simulink model "rawread_slx"  (R2023b)
settings: Solver=FixedStepAuto  StartTime=0.0  StopTime=0  RelTol=1e-3
values from neighbouring files (symbols this model uses):
  m = zeros(size(cfa, 1), 1)    [do.m]
  n = zeros(size(cfa, 2), 1)    [do.m]
  wb = rawInfo.ColorInfo.CameraAsTakenWhiteBalance    [do.m]
  wbcam = rawInfo.ColorInfo.D65WhiteBalance    [do.m]
  xyz = rawInfo.ColorInfo.CameraToXYZ    [do.m]
undefined symbols (not defined in the file or in its folder): gray
settings Model: ParamWorkspaceSource=ReferencedWorkspace  Creator=49176  LastModifiedBy=vithani
settings SolverCC: AllowMultiTaskInputOutput=on  ConcurrentTasks=on  AutoInsertRateTranBlk=on
settings SFSimCC: SimTargetLang=C++

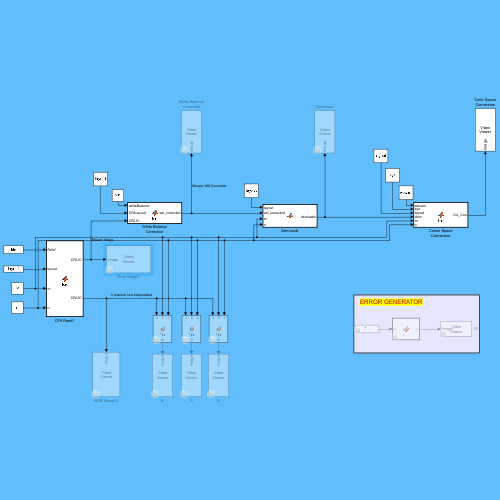
[thumbnail: Simulink's stored preview of the top-level diagram]
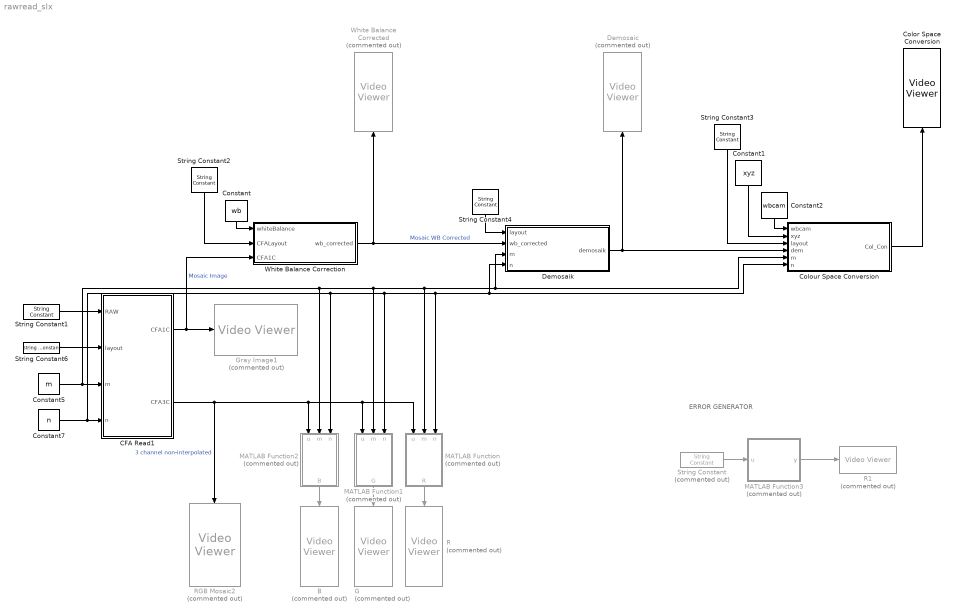
== system rawread_slx ==
  note: ERROR GENERATOR
  B : VideoViewer  Commented=on  colormapValue=gray(256)  FigPos=[1003 1173.33333333333 826.666666666667 737.333333333333]
  CFA Read1 : MATLAB Function  TreatAsAtomicUnit=on
  Color Space Conversion : VideoViewer  colormapValue=gray(256)  FigPos=[771.666666666667 1071.33333333333 884 518]
  Colour Space Conversion : MATLAB Function  TreatAsAtomicUnit=on
  Constant : Constant  Value=wb
  Constant1 : Constant  Value=xyz
  Constant2 : Constant  Value=wbcam
  Constant5 : Constant  Value=m  VectorParams1D=off
  Constant7 : Constant  Value=n  VectorParams1D=off
  Demosaic : VideoViewer  Commented=on  colormapValue=gray(256)  FigPos=[715.666666666667 964 852 619.333333333333]
  Demosaik : MATLAB Function  TreatAsAtomicUnit=on
  G : VideoViewer  Commented=on  colormapValue=gray(256)  FigPos=[819.666666666667 1044.66666666667 714 319.333333333333]
  Gray Image1 : VideoViewer  Commented=on  colormapValue=gray(256)  FigPos=[423 1558.66666666667 1238.66666666667 816.666666666667]
  MATLAB Function : MATLAB Function  Commented=on  TreatAsAtomicUnit=on
  MATLAB Function1 : MATLAB Function  Commented=on  TreatAsAtomicUnit=on
  MATLAB Function2 : MATLAB Function  Commented=on  TreatAsAtomicUnit=on
  MATLAB Function3 : MATLAB Function  Commented=on  TreatAsAtomicUnit=on
  R : VideoViewer  Commented=on  colormapValue=gray(256)  FigPos=[881 962 798.666666666667 486]
  R1 : VideoViewer  Commented=on  colormapValue=gray(256)  FigPos=[881 962 798.666666666667 486]
  RGB Mosaic2 : VideoViewer  Commented=on  colormapValue=gray(256)  FigPos=[924.333333333333 1074.66666666667 930 472]
  String Constant : StringConstant  Commented=on  String=file
  String Constant1 : StringConstant  String=file
  String Constant{2..4,6} (4 alike) : StringConstant  String=layout
  White Balance Corrected : VideoViewer  Commented=on  colormapValue=gray(256)  FigPos=[1323.66666666667 1579.33333333333 958.666666666667 1055.33333333333]
  White Balance Correction : MATLAB Function  TreatAsAtomicUnit=on
  wires:
  CFA Read1/1(CFA1C) -> White Balance Correction/3(CFA1C), Gray Image1/1  "Mosaic Image"
  String Constant1/1 -> CFA Read1/1(RAW)
  CFA Read1/2(CFA3C) -> MATLAB Function/1(u), MATLAB Function1/1(u), MATLAB Function2/1(u), RGB Mosaic2/1  "3 channel non-interpolated"
  MATLAB Function/1(R) -> R/1
  MATLAB Function1/1(G) -> G/1
  MATLAB Function2/1(B) -> B/1
  White Balance Correction/1(wb_corrected) -> White Balance Corrected/1, Demosaik/2(wb_corrected)  "Mosaic WB Corrected"
  Colour Space Conversion/1(Col_Con) -> Color Space Conversion/1
  Constant/1 -> White Balance Correction/1(whiteBalance)
  String Constant2/1 -> White Balance Correction/2(CFALayout)
  Demosaik/1(demosaik) -> Demosaic/1, Colour Space Conversion/4(dem)
  Constant2/1 -> Colour Space Conversion/1(wbcam)
  Constant1/1 -> Colour Space Conversion/2(xyz)
  String Constant3/1 -> Colour Space Conversion/3(layout)
  String Constant4/1 -> Demosaik/1(layout)
  String Constant6/1 -> CFA Read1/2(layout)
  Constant5/1 -> CFA Read1/3(m), MATLAB Function1/2(m), Colour Space Conversion/5(m), Demosaik/3(m), MATLAB Function/2(m), MATLAB Function2/2(m)
  Constant7/1 -> MATLAB Function/3(n), Colour Space Conversion/6(n), Demosaik/4(n), MATLAB Function1/3(n), MATLAB Function2/3(n), CFA Read1/4(n)
  MATLAB Function3/1(y) -> R1/1
  String Constant/1 -> MATLAB Function3/1(u)

== matlab function rawread_slx/CFA Read1 ==
  data: RAW input; CFA1C output; CFA3C output; layout input; m input; n input
function [CFA1C, CFA3C] = fcn(RAW, layout, m, n)

% to mitigate code generation error as limitaion with simulink fcn block
coder.extrinsic("rawread", "rawinfo", "imfinfo","im2uint16");

% global var
a = size(m, 1) ; b = size(n, 1);

% pre-initialising
cfa     = zeros(a, b, "double");
red     = zeros(a, b, "uint16");
blue    = zeros(a, b, "uint16");
green   = zeros(a, b, "uint16");
R       = zeros(a, b, "uint16");
G       = zeros(a, b, "uint16");
B       = zeros(a, b, "uint16");

% raw read and metadata
imgInfo1        = rawinfo(RAW);
imgInfo1        = imfinfo(RAW);
cfa             = im2double(rawread(RAW));


% CFA1C out; default matlab fcn
CFA1C = zeros(a, b, "uint16");

%{--------------- CFA3C begin ---------------%}
% CFA3C algo

i = a; j = b;
red = cfa;
blue = cfa;
green = cfa;

if layout == "RGGB"
    % RED
    for x = 1:i
        even = mod(x,2);
        if even == 0
            red(x, :) = NaN;
        end
    end
    for y = 1:j
        even = mod(y,2);
        if even == 0
            red(:, y) = NaN;
        end
    end
    % BLUE
    for x = 1:i
        even = mod(x, 2);
        if even == 1
            blue(x, :) = NaN;
        end
    end
    for y = 1:j
        even = mod(y, 2);
        if even == 1
            blue(:, y) = NaN;
        end
    end
    % GREEN
    for x = 1:i
        even = mod(x, 2);
        if even == 1
            for y = 1:j
                even = mod(y,2);
                if even == 1
                    green(x, y) = NaN;
                end
            end
        end
        even = mod(x, 2);
        if even ~= 1
            for y = 1:j
                even = mod(y, 2);
                if even == 0
                    green(x, y) = NaN;
                end
            end
        end
    end
end

if layout == "BGGR"
    % RED
    for x = 1:i
        even = mod(x,2);
        if even == 0
            red(x, :) = NaN;
        end
    end
    for y = 1:j
        even = mod(y,2);
        if even == 0
            red(:, y) = NaN;
        end
    end
    % BLUE
    for x = 1:i
        even = mod(x, 2);
        if even == 1
            blue(x, :) = NaN;
        end
    end
    for y = 1:j
        even = mod(y, 2);
        if even == 1
            blue(:, y) = NaN;
        end
    end
    % GREEN
    for x = 1:i
        even = mod(x, 2);
        if even == 1
            for y = 1:j
                even = mod(y,2);
                if even == 1
                    green(x, y) = NaN;
                end
            end
        end
        even = mod(x, 2);
        if even ~= 1
            for y = 1:j
                even = mod(y, 2);
                if even == 0
                    green(x, y) = NaN;
                end
            end
        end
    end
end


if layout == "GRBG"
    % RED
    for x = 1:i
        even = mod(x, 2);
        if even ~= 1
            red(x, :) = NaN;
        end
    end
    for y = 1:j
        even = mod(y, 2);
        if even == 1
            red(:, y) = NaN;
        end
    end

    % BLUE
    for x = 1:i
        even = mod(x, 2);
        if even ~= 0
            blue(x, :) = NaN;
        end
    end
    for y = 1:j
        even = mod(y, 2);
        if even == 0
            blue(:, y) = NaN;
        end
    end
    % GREEN
    for x = 1:i
        even = mod(x, 2);
        if even == 1
            for y = 1:j
                even = mod(y, 2);
                if even ~= 1
                    green(x, y) = NaN;
                end
            end
        end
        even = mod(x, 2);
        if even ~= 1
            for y = 1:j
                even = mod(y, 2);
                if even ~= 0
                    green(x, y) = NaN;
                end
            end
        end
    end
end

if layout == "GBRG"
    % RED
    for x = 1:i
        even = mod(x, 2);
        if even ~= 1
            red(x, :) = NaN;
        end
    end
    for y = 1:j
        even = mod(y, 2);
        if even == 1
            red(:, y) = NaN;
        end
    end

    % BLUE
    for x = 1:i
        even = mod(x, 2);
        if even ~= 0
            blue(x, :) = NaN;
        end
    end
    for y = 1:j
        even = mod(y, 2);
        if even == 0
            blue(:, y) = NaN;
        end
    end
    % GREEN
    for x = 1:i
        even = mod(x, 2);
        if even == 1
            for y = 1:j
                even = mod(y, 2);
                if even ~= 1
                    green(x, y) = NaN;
                end
            end
        end
        even = mod(x, 2);
        if even ~= 1
            for y = 1:j
                even = mod(y, 2);
                if even ~= 0
                    green(x, y) = NaN;
                end
            end
        end
    end
end

% preinitialization
CFA3C = zeros(a, b, 3, "uint16");

CFA3C(:,:,1)=im2uint16(red);
CFA3C(:,:,2)=im2uint16(green);
CFA3C(:,:,3)=im2uint16(blue);

%{--------------- CFA3C end ---------------%}


% output ports
CFA1C = im2uint16(cfa);

== matlab function rawread_slx/MATLAB Function3 ==
  data: u input; y output; A data_store_memory; B data_store_memory
function y = fcn(u)
global A B;
coder.extrinsic('rawread')
y = zeros(2638, 3920, 'uint16')
y = rawread(u);

== matlab function rawread_slx/MATLAB Function ==
  data: u input; R output; m input; n input
function R = fcn(u, m, n)

a = size(m, 1); b = size(n, 1);

R = zeros(a, b, 3, 'uint16');
R(:, :, 1) = u(:, :, 1);

== matlab function rawread_slx/MATLAB Function1 ==
  data: u input; G output; m input; n input
function G = fcn(u, m, n)

a = size(m, 1); b = size(n, 1);

G = zeros(a, b, 3,'uint16');
G(: ,:, 2) = u(:, :, 2);

== matlab function rawread_slx/MATLAB Function2 ==
  data: u input; B output; m input; n input
function B = fcn(u, m, n)

a = size(m, 1); b = size(n, 1);

B = zeros(a, b, 3, 'uint16');
B(:, :, 3) = u(:, :, 3);

== matlab function rawread_slx/Demosaik ==
  data: layout input; wb_corrected input; demosaik output; m input; n input
function demosaik = fcn(layout, wb_corrected, m, n)

% preinitialization




%{--------------- CFA3C BEGIN ---------------%}
% CFA3C algo
wb_corrected = im2double(wb_corrected)

i = size(m, 1); j = size(n, 1);
% i = m; j = n;

red = wb_corrected;
blue = wb_corrected;
green = wb_corrected;


if layout == "RGGB"
    % RED
    for x = 1:i
        even = mod(x,2);
        if even == 0
            red(x, :) = NaN;
        end
    end
    for y = 1:j
        even = mod(y,2);
        if even == 0
            red(:, y) = NaN;
        end
    end
    % BLUE
    for x = 1:i
        even = mod(x, 2);
        if even == 1
            blue(x, :) = NaN;
        end
    end
    for y = 1:j
        even = mod(y, 2);
        if even == 1
            blue(:, y) = NaN;
        end
    end
    % GREEN
    for x = 1:i
        even = mod(x, 2);
        if even == 1
            for y = 1:j
                even = mod(y,2);
                if even == 1
                    green(x, y) = NaN;
                end
            end
        end
        even = mod(x, 2);
        if even ~= 1
            for y = 1:j
                even = mod(y, 2);
                if even == 0
                    green(x, y) = NaN;
                end
            end
        end
    end
end

if layout == "BGGR"
    % RED
    for x = 1:i
        even = mod(x,2);
        if even == 0
            red(x, :) = NaN;
        end
    end
    for y = 1:j
        even = mod(y,2);
        if even == 0
            red(:, y) = NaN;
        end
    end
    % BLUE
    for x = 1:i
        even = mod(x, 2);
        if even == 1
            blue(x, :) = NaN;
        end
    end
    for y = 1:j
        even = mod(y, 2);
        if even == 1
            blue(:, y) = NaN;
        end
    end
    % GREEN
    for x = 1:i
        even = mod(x, 2);
        if even == 1
            for y = 1:j
                even = mod(y,2);
                if even == 1
                    green(x, y) = NaN;
                end
            end
        end
        even = mod(x, 2);
        if even ~= 1
            for y = 1:j
                even = mod(y, 2);
                if even == 0
                    green(x, y) = NaN;
                end
            end
        end
    end
end


if layout == "GRBG"
    % RED
    for x = 1:i
        even = mod(x, 2);
        if even ~= 1
            red(x, :) = NaN;
        end
    end
    for y = 1:j
        even = mod(y, 2);
        if even == 1
            red(:, y) = NaN;
        end
    end

    % BLUE
    for x = 1:i
        even = mod(x, 2);
        if even ~= 0
            blue(x, :) = NaN;
        end
    end
    for y = 1:j
        even = mod(y, 2);
        if even == 0
            blue(:, y) = NaN;
        end
    end
    % GREEN
    for x = 1:i
        even = mod(x, 2);
        if even == 1
            for y = 1:j
                even = mod(y, 2);
                if even ~= 1
                    green(x, y) = NaN;
                end
            end
        end
        even = mod(x, 2);
        if even ~= 1
            for y = 1:j
                even = mod(y, 2);
                if even ~= 0
                    green(x, y) = NaN;
                end
            end
        end
    end
end

if layout == "GBRG"
    % RED
    for x = 1:i
        even = mod(x, 2);
        if even ~= 1
            red(x, :) = NaN;
        end
    end
    for y = 1:j
        even = mod(y, 2);
        if even == 1
            red(:, y) = NaN;
        end
    end

    % BLUE
    for x = 1:i
        even = mod(x, 2);
        if even ~= 0
            blue(x, :) = NaN;
        end
    end
    for y = 1:j
        even = mod(y, 2);
        if even == 0
            blue(:, y) = NaN;
        end
    end
    % GREEN
    for x = 1:i
        even = mod(x, 2);
        if even == 1
            for y = 1:j
                even = mod(y, 2);
                if even ~= 1
                    green(x, y) = NaN;
                end
            end
        end
        even = mod(x, 2);
        if even ~= 1
            for y = 1:j
                even = mod(y, 2);
                if even ~= 0
                    green(x, y) = NaN;
                end
            end
        end
    end
end


%{--------------- CFA3C END ---------------%}


%{--------------- DEMOSAIC BEGIN ---------------%}

img_mosaik = zeros(i, j, 3);
img_mosaik = zeros(i, j, 3);
img_mosaik = zeros(i, j, 3);
img_mosaik(:, :, 1) = red;
img_mosaik(:, :, 2) = green;
img_mosaik(:, :, 3) = blue;
demosaik = img_mosaik;

for x = 2:(i - 2)
    for y = 2:(j - 2)
        if isnan(demosaik(x, y, 1))
            demosaik(x, y, 1) = (demosaik(x, y - 1, 1) + demosaik(x, y + 1, 1)) / 2;
        end
    end
end
for x = 2:(i - 2)
    for y = 1:(j - 2)
        if isnan(demosaik(x, y, 1))
            demosaik(x, y, 1) = (demosaik(x - 1, y, 1)+demosaik(x + 1, y, 1)) / 2;
        end
    end
end

for x = 2:(i - 2)
    for y = 2:(j - 2)
        if isnan(demosaik(x, y, 2))
            demosaik(x, y, 2) = (demosaik(x - 1, y, 2) + demosaik(x, y - 1, 2) + demosaik(x, y + 1, 2) + demosaik(x + 1, y, 2)) / 4;
        end
    end
end

for x = 2:(i - 2)
    for y = 2:(j - 2)
        if isnan(demosaik(x, y, 3))
            demosaik(x, y, 3) = (demosaik(x, y - 1, 3) + demosaik(x, y + 1, 3)) / 2;
        end
    end
end
for x = 2:(i - 2)
    for y = 2:(j - 2)
        if isnan(demosaik(x, y, 3))
            demosaik(x, y, 3) = (demosaik(x-1, y, 3) + demosaik(x + 1, y, 3)) / 2;
        end
    end
end

if contains(layout, "BGGR")
    allo1 = demosaik(:, :, 1);
    allo3 = demosaik(:, :, 3);
    demosaik(:, :, 1) = allo3;
    demosaik(:, :, 3) = allo1;
end
if contains(layout, "GBRG")
    allo1 = demosaik(:, :, 1);
    allo3 = demosaik(:, :, 3);
    demosaik(:, :, 1) = allo3;
    demosaik(:, :, 3) = allo1;
end

%{--------------- DEMOSAIC END ---------------%}

== matlab function rawread_slx/White Balance Correction ==
  data: whiteBalance input; CFALayout input; wb_corrected output; CFA1C input
function wb_corrected = fcn(whiteBalance, CFALayout, CFA1C)

coder.extrinsic("rawinfo")

% wb as green channel
gLoc = strfind(CFALayout,"G");
gLoc = gLoc(1);

% CFA1C feature scaling / normalization
CFA1C = double(CFA1C)
maxValue = max(CFA1C(:))
CFA1C = CFA1C ./ maxValue


% wb array construction
whiteBalance = whiteBalance/whiteBalance(gLoc);
whiteBalance = reshape(whiteBalance,2,2)
dim = size(CFA1C)./size(whiteBalance)
whiteBalance = repmat(whiteBalance,dim)

% wb array dot-product with CFA1C
CFA1C = im2uint16(CFA1C.* whiteBalance)

% output
wb_corrected = CFA1C;

== matlab function rawread_slx/Colour Space Conversion ==
  data: wbcam input; xyz input; layout input; dem input; Col_Con output; m input; n input
function Col_Con = fcn(wbcam, xyz, layout, dem, m, n)

coder.extrinsic("imapplymatrix","xyz2rgb");

i = size(m, 1); j = size(n, 1);
% pre-initalizing
Col_Con = zeros(i, j, 3, "uint16");
wbIdx = zeros(1, 3)


wbIdx(1) = strfind(layout,"R")
gidx = strfind(layout,"G")
wbIdx(2) = gidx(1)
wbIdx(3) = strfind(layout,"B")

wbcam = wbcam'
wbCoeffs = wbcam(wbIdx)
xyz = xyz ./ wbCoeffs

imXYZ = imapplymatrix(xyz, im2double(dem));
Col_Con = xyz2rgb(imXYZ, OutputType="uint16");
